simulink model "navigation"  (R2023b)
settings: Solver=ode45  StartTime=0.0  StopTime=28.2  MaxStep=0.00005  RelTol=1e-12  AbsTol=1e-12
values from neighbouring files (symbols this model uses):
  distance_between_wheels = 0.5    [main.m]
  wheel_radius = 0.01    [main.m]
settings Model: Creator=kai  LastModifiedBy=anderstai

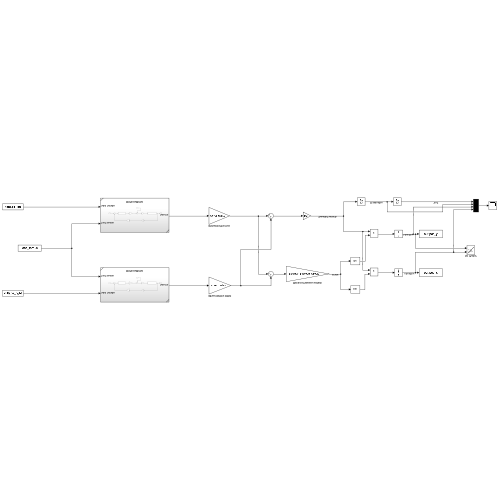
[thumbnail: Simulink's stored preview of the top-level diagram]
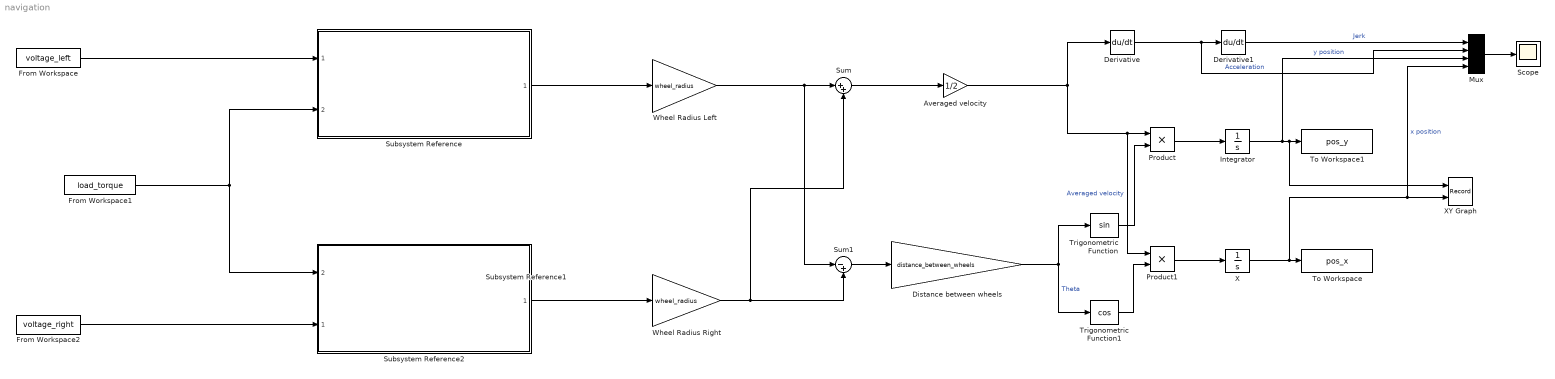
== system navigation ==
  Averaged velocity : Gain  Gain=1/2
  Derivative : Derivative
  Derivative1 : Derivative
  Distance between wheels : Gain  Gain=distance_between_wheels
  From Workspace : FromWorkspace  VariableName=voltage_left
  From Workspace1 : FromWorkspace  VariableName=load_torque
  From Workspace2 : FromWorkspace  VariableName=voltage_right
  Integrator : Integrator
  Mux : Mux
  Product : Product
  Product1 : Product
  Scope : Scope
  Subsystem Reference : Subsystem  ReferencedSubsystem=DCMotorModel
  Subsystem Reference1 : Subsystem  ReferencedSubsystem=<file name>
  Subsystem Reference2 : Subsystem  ReferencedSubsystem=DCMotorModel
      settings: PortSchema="{\"entries\":[{\"content\":{\"sides\":[{\"content\":{\"connectorIds\":[\"In2\",\"In1\"]},\"type\":\"ConnectorPlacement.EquallySpacedRectSide\",\"uuid\":\"01d996e7-ae2d-4523-b6ce-507f81d0b027\"},{\"content\":{\"connectorIds\":[\"Out1\"],\"side\":\"RIGHT\"},\"type\":\"ConnectorPlacement.EquallySpacedRectSide\",\"uuid\":\"ad13a777-31d0-47d6-89de-a80db1c69617\"},{\"content\":{\"side\":\"TOP\"},\"type\":\"ConnectorPlacement.EquallySpacedRectSide\",\"uuid\":\"6a617c68-c41c-4df7-956e-9625de4178d9\"}]},\"type\":\"ConnectorPlacement.EquallySpacedConnector\",\"uuid\":\"7d3c3038-80a4-415c-9373-7ed211e56de6\"}],\"packageUris\":[\"http://schema.mathworks.com/mf0/Connector/R2020b\"],\"version\":\"1.0\"}"
  Sum : Sum  Inputs=|++
  Sum1 : Sum  Inputs=|-+
  To Workspace : ToWorkspace  VariableName=pos_x  SaveFormat=Timeseries  SampleTime=-1
  To Workspace1 : ToWorkspace  VariableName=pos_y  SaveFormat=Timeseries  SampleTime=-1
  Trigonometric Function : Trigonometry
  Trigonometric Function1 : Trigonometry  Operator=cos
  Wheel Radius Left : Gain  Gain=wheel_radius
  Wheel Radius Right : Gain  Gain=wheel_radius
  X : Integrator
  XY Graph : Record  FileSettingsInternal="{\"entries\":[{\"content\":{\"excelSettings\":{\"content\":{},\"type\":\"Streamout.ExcelSettings\"}},\"type\":\"Streamout.FileSettingStorage\",\"uuid\":\"\"}],\"packageUris\":[\"http:\\/\\/schema.mathworks.com\\/mf0\\/streamout_blocks\\/R2020a\"],\"version\":\"1.0\"}"  Layout=[1 1]  SignalsInternal="{\"entries\":[{\"content\":{\"signals\":[{\"content\":{\"blockPath\":[],\"dimensions\":[1],\"domain\":\"\",\"lineColor\":\"#a2142f\",\"plots\":[1],\"port\":1,\"signalID\":40,\"signalName\":\"XY Graph:1\"},\"type\":\"RecordBlkView.Signal\",\"uuid\":\"\"},{\"content\":{\"blockPath\":[],\"dimensions\":[1],\"domain\":\"\",\"lineColor\":\"#139fff\",\"plots\":[1],\"port\":2,\"signalID\":43,\"signalName\":\"XY Graph:2\"},\"type\":\"RecordBlkView.Signal\",\"uuid\":\"\"}]},\"type\":\"RecordBlkView.InputSignals\",\"uuid\":\"\"}],\"packageUris\":[\"http:\\/\\/schema.mathworks.com\\/mf0\\/streamout_blocks\\/R2020a\"],\"version\":\"1.0\"}"  VisualizationBindings="{\"xyplotplugin\":{\"info\":[{\"series\":[{\"bindingParametersList\":[{\"parameter\":\"X-Axis\",\"signalID\":40,\"signalName\":\"XY Graph:1\"},{\"parameter\":\"Y-Axis\",\"signalID\":43,\"signalName\":\"XY Graph:2\"}],\"seriesID\":38237}],\"subplotID\":1}]}}"  CompatibilityTag=XY  st=-1
  wires:
  From Workspace1/1 -> Subsystem Reference2/2, Subsystem Reference/2
  Subsystem Reference2/1 -> Wheel Radius Right/1
  Subsystem Reference/1 -> Wheel Radius Left/1
  Wheel Radius Left/1 -> Sum1/1, Sum/1
  Wheel Radius Right/1 -> Sum1/2, Sum/2
  Sum/1 -> Averaged velocity/1
  Sum1/1 -> Distance between wheels/1
  Distance between wheels/1 -> Trigonometric Function1/1, Trigonometric Function/1  "Theta"
  Trigonometric Function/1 -> Product/2
  Averaged velocity/1 -> Product/1, Product1/1, Derivative/1  "Averaged velocity"
  Product/1 -> Integrator/1
  Trigonometric Function1/1 -> Product1/2
  Product1/1 -> X/1
  X/1 -> Mux/4, XY Graph/2, To Workspace/1  "x position"
  Integrator/1 -> Mux/3, XY Graph/1, To Workspace1/1  "y position"
  Derivative/1 -> Mux/2, Derivative1/1  "Acceleration"
  Derivative1/1 -> Mux/1  "Jerk"
  Mux/1 -> Scope/1
  From Workspace2/1 -> Subsystem Reference2/1
  From Workspace/1 -> Subsystem Reference/1

== system navigation/Subsystem Reference1 ==
